simulink model "Shock_sim"  (R2016b)
settings: Solver=ode4  StartTime=0.0  StopTime=tfin  FixedStep=1e-5  RelTol=1e-3
values from neighbouring files (symbols this model uses):
  lamb1 = om_xy(1)    [main.m]
  Ry = fi_xy.'*M_xy*delta_y    [main.m]
undefined symbols (not defined in the file or in its folder): fi_xy, sigbuilder_block
settings Model: Creator=Salvo  LastModifiedBy=Salvo

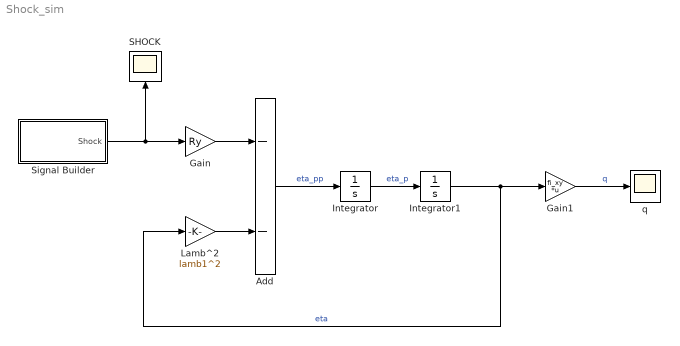
== system Shock_sim ==
  Add : Sum  Inputs=--
  Gain : Gain  Gain=Ry
  Gain1 : Gain  Gain=fi_xy  Multiplication=Matrix(K*u)
  Integrator : Integrator
  Integrator1 : Integrator
  Lamb^2 : Gain  Gain=lamb1^2
  SHOCK : Scope
  Signal Builder : Subsystem  Tag=STV Subsys  LoadFcn=sigbuilder_block('load');  StartFcn=sigbuilder_block('start');  StopFcn=sigbuilder_block('stop');  ClipboardFcn=sigbuilder_block('clipboard');  mask(Sigbuilder block){tuvar=[0:10]}
      mask help: Simulink:masks:SigbuilderBlock_MD
      mask init:
      | if ~strcmp(get_param(bdroot(gcbh),'SimulationStatus'),'stopped') tuvar = sigbuilder_block('maskInit'); end
      settings: CopyFcn=sigbuilder_block('copy');  DeleteFcn=sigbuilder_block('delete');  ModelCloseFcn=sigbuilder_block('modelClose');  PreSaveFcn=sigbuilder_block('preSave');  PauseFcn=sigbuilder_block('pause');  ContinueFcn=sigbuilder_block('continue');  NameChangeFcn=sigbuilder_block('namechange');  OpenFcn=sigbuilder_block('open',[437.25 153 550.5 359.25 ]);  CloseFcn=sigbuilder_block('close');
      mask Display: plot(0, 0, 100, 100,[2, 2, 32, 32, 2], [68, 8, 8, 68, 68],[32, 2], [38, 38], [32, 19, 2],[53, 60, 44], [32, 17, 17, 2],[16, 16, 31, 31]);txt = getActiveGroup(gcbh);text(2, 100, txt,'verticalAlignment', 'top');
  q : Scope
  wires:
  Signal Builder/1(Shock) -> Gain/1, SHOCK/1
  Gain/1 -> Add/1
  Add/1 -> Integrator/1  "eta_pp"
  Integrator/1 -> Integrator1/1  "eta_p"
  Integrator1/1 -> Gain1/1, Lamb^2/1  "eta"
  Lamb^2/1 -> Add/2
  Gain1/1 -> q/1  "q"

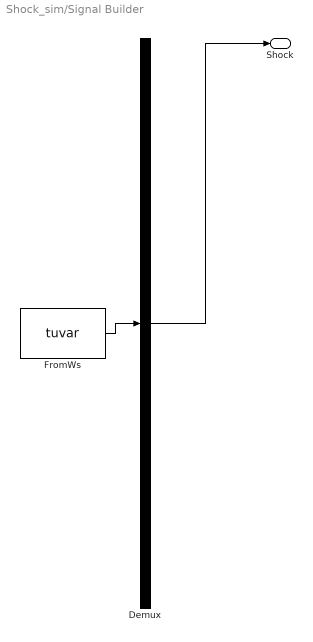
== system Shock_sim/Signal Builder ==
  Demux : Demux  Tag=STV Demux  Outputs=1
  FromWs : FromWorkspace  Tag=STV FromWs  VariableName=tuvar  SampleTime=0
      SigBuilderData=|
      | common.afterFinalStr = 'Extrapolate'
      | common.sampleTime = 0
      | dataSet.timeRange = [0 10]
      | dataSet.name = 'Group 1'
      | sbobj.Groups.Name = 'Group 1'
      | sbobj.Groups.Signals.Name = 'Shock'
      | sbobj.Groups.Signals.XData = [0 0.011 0.011 10]
      | sbobj.Groups.Signals.YData = [0 196.2 0 0]
  Shock : Outport  Tag=STV Outport
  wires:
  Demux/1 -> Shock/1
  FromWs/1 -> Demux/1
